simulink model "sst_cllc_ttype_inv"  (R2026a)
settings: Solver=ode23tb  StopTime=simlength  FixedStep=tc  MaxStep=glb_time.tc
values from neighbouring files (symbols this model uses):
  afe_ctrl = ctrl_afe_setup(glb_time.ts_afe, grid_emu.omega_grid_nom)    [init_model.m]
  cllc_ctrl = ctrl_cllc_setup(kp_udc, ki_udc, kp_idc, ki_idc)    [init_model.m]
  glb_time = timing_setup(fpwm_afe, trgo_afe, fpwm_inv, trgo_inv, fpwm_single_phase_inv, trgo_single_phase_inv, fpwm_dab, trgo_dab,      fpwm_psfbc, trgo_psfbc, fpwm_isop_rail, trgo_isop_rail, fpwm_cllc, trgo_cllc, t_measure, tc_factor, tc_decimation, delay_pwm, dead_time_afe,      dead_time_inv, dead_time_single_phase_inv, dead_time_dab, dead_time_psfbc, dead_time_isop_rail, dead_time_cllc)    [init_model.m]
  grid_emu = grid_three_phase_emulator('Dyn11', delta_star, grid_nominal_power, application_voltage, us1, us2, fgrid,                  eq_grid_inductance, eq_grid_resistance, eta, ucc, i1m, p_iron, n1, n2, core_area, core_length, mur,                  up_xi_pu_ref, up_eta_pu_ref, un_xi_pu_ref, un_eta_pu_ref)    [init_model.m]
  lithium_ion_battery_1 = lithium_ion_battery_setup(nominal_battery_voltage_1, nominal_battery_power, initial_battery_soc, glb_time.ts_dab)    [init_model.m]
  omega_set = frequency_set*2*pi    (= 1884.95559215)    [init_model.m]
  single_phase_inverter_ctrl = ctrl_single_phase_inverter_setup(glb_time.ts_inv, pres_ctrl.omega_set,      dqvector_pi.kp_inv, dqvector_pi.ki_inv, pres_ctrl.kp_rpi, pres_ctrl.ki_rpi, pres_ctrl.delta_rpi)    [init_model.m]
  sst_num_of_modules = 2    [init_model.m]
undefined symbols (not defined in the file or in its folder): hwdata
libraries: fl_lib x62, nesl_utility x38, discrete_time_low_pass_filter x8, full_bridge_ideal_switch x4, full_bridge_mosfet_based_with_thermal_model x4, full_bridge_mosfet_based_with_thermal_model_zvs x4, lithium_ion_battery x2, single_phase_transformer x2, dab_single_phase_pwm_modulator x2, dclink_for_three_levels x2, full_bridge_three_level_ttype_ideal_switch_based_model x2, full_bridge_three_level_ttype_mosfet_based_model x2
(part 3 of 5)

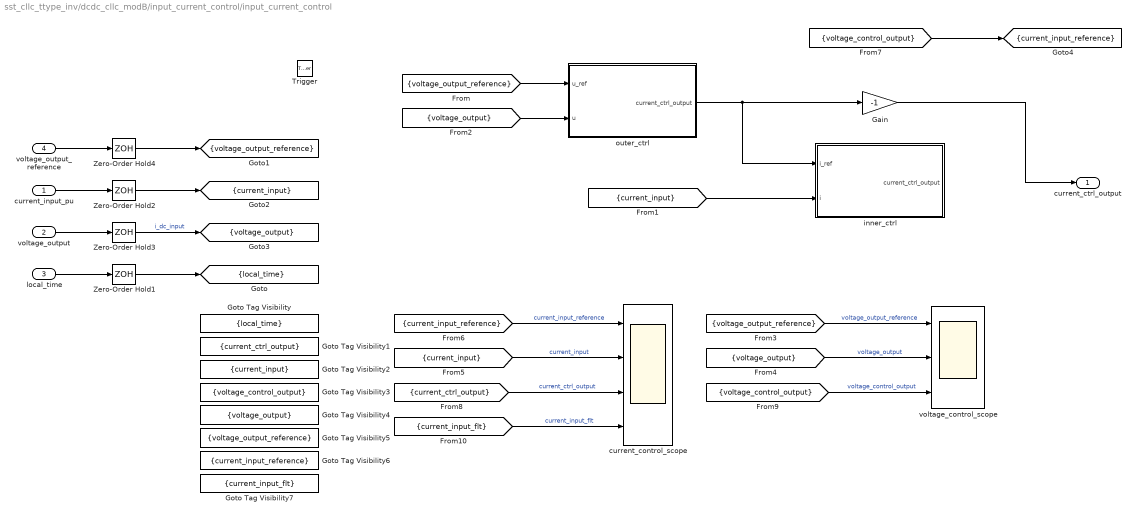
== system sst_cllc_ttype_inv/dcdc_cllc_modB/input_current_control/input_current_control ==
  current_input_pu : Inport
  voltage_output : Inport  Port=2
  local_time : Inport  Port=3
  voltage_output_reference : Inport  Port=4
  Trigger : TriggerPort  VariantControl=(inherit)  PortDimensions=1
  Gain : Gain  Gain=-1
  Goto Tag Visibility : GotoTagVisibility  GotoTag=local_time
  Goto Tag Visibility1 : GotoTagVisibility  GotoTag=current_ctrl_output
  Goto Tag Visibility2 : GotoTagVisibility  GotoTag=current_input
  Goto Tag Visibility3 : GotoTagVisibility  GotoTag=voltage_control_output
  Goto Tag Visibility4 : GotoTagVisibility  GotoTag=voltage_output
  Goto Tag Visibility5 : GotoTagVisibility  GotoTag=voltage_output_reference
  Goto Tag Visibility6 : GotoTagVisibility  GotoTag=current_input_reference
  Goto Tag Visibility7 : GotoTagVisibility  GotoTag=current_input_flt
  Zero-Order Hold{1..4} (4 alike) : ZeroOrderHold  SampleTime=-1
  current_control_scope : Scope  NumInputPorts=4
      settings: ActiveDisplayYMinimum=-0.89123984985351878  ActiveDisplayYMaximum=0.96302534790039185  DataLoggingVariableName=ScopeData12
  inner_ctrl : Subsystem
  outer_ctrl : Subsystem
  voltage_control_scope : Scope  NumInputPorts=3
      settings: ActiveDisplayYMinimum=-2.2572021484375  ActiveDisplayYMaximum=10.3148193359375  DataLoggingVariableName=ScopeData7
  current_ctrl_output : Outport
  tag scope: current_input=scoped, current_input_reference=scoped, local_time=scoped, voltage_output=scoped, voltage_output_reference=scoped
  wires:
  [current_input_flt] -> current_control_scope/4  "current_input_flt"
  [voltage_control_output] -> voltage_control_scope/3  "voltage_control_output"
  [voltage_output] -> voltage_control_scope/2  "voltage_output"
  [voltage_output_reference] -> voltage_control_scope/1  "voltage_output_reference"
  [current_ctrl_output] -> current_control_scope/3  "current_ctrl_output"
  [voltage_control_output] -> [current_input_reference]
  [current_input_reference] -> current_control_scope/1  "current_input_reference"
  [current_input] -> current_control_scope/2  "current_input"
  [voltage_output] -> outer_ctrl/2(u)
  [current_input] -> inner_ctrl/2(i)
  outer_ctrl/1(current_ctrl_output) -> Gain/1, inner_ctrl/1(i_ref)
  [voltage_output_reference] -> outer_ctrl/1(u_ref)
  Zero-Order Hold3/1 -> [voltage_output]  "i_dc_input"
  Zero-Order Hold2/1 -> [current_input]
  Zero-Order Hold4/1 -> [voltage_output_reference]
  voltage_output_reference/1 -> Zero-Order Hold4/1
  Zero-Order Hold1/1 -> [local_time]
  voltage_output/1 -> Zero-Order Hold3/1
  local_time/1 -> Zero-Order Hold1/1
  current_input_pu/1 -> Zero-Order Hold2/1
  Gain/1 -> current_ctrl_output/1

== system sst_cllc_ttype_inv/dcdc_cllc_modB/input_current_control/modulator ==
  phase_displacement : Inport
  Constant1 : Constant  Value=0.5
  Constant2 : Constant  Value=0.5
  dab_single_phase_pwm_modulator : dab_single_phase_pwm_modulator/dab_single_phase_pwm_modulator  fPWM_DAB=glb_time.fPWM_CLLC  m_up=1  m_low=0  dead_time_DAB=glb_time.dead_time_CLLC  pos_cmd_gate=18  neg_cmd_gate=-3  polarity=-1  tc=glb_time.tc  max_phase_displacement=pi/2  trgo_double_update=glb_time.TRGO_CLLC_double_update
  gate_cmds : Outport
  tag scope: TRGO_cllc_modB=global
  wires:
  phase_displacement/1 -> dab_single_phase_pwm_modulator/4
  [time_cllc_module_B] -> dab_single_phase_pwm_modulator/1
  Constant1/1 -> dab_single_phase_pwm_modulator/2
  dab_single_phase_pwm_modulator/1 -> [TRGO_cllc_modB]
  Constant2/1 -> dab_single_phase_pwm_modulator/3
  dab_single_phase_pwm_modulator/2 -> gate_cmds/1

== system sst_cllc_ttype_inv/dcdc_cllc_modB/input_current_control/normalization ==
  in : Inport
  1/Ti3 : Gain  Gain=1/hwdata.cllc.idc1_bez  OutDataTypeStr=double  SaturateOnIntegerOverflow=on  ParamDataTypeStr=Inherit: Same as input
  Quantizer : Quantizer  QuantizationInterval=adc12_quantization
  out_pu : Outport
  wires:
  Quantizer/1 -> out_pu/1
  1/Ti3/1 -> Quantizer/1
  in/1 -> 1/Ti3/1

== system sst_cllc_ttype_inv/dcdc_cllc_modB/input_current_control/normalization1 ==
  in : Inport
  1/Ti3 : Gain  Gain=1/hwdata.cllc.udc2_bez  OutDataTypeStr=double  SaturateOnIntegerOverflow=on  ParamDataTypeStr=Inherit: Same as input
  Quantizer : Quantizer  QuantizationInterval=adc12_quantization
  out_pu : Outport
  wires:
  Quantizer/1 -> out_pu/1
  in/1 -> 1/Ti3/1
  1/Ti3/1 -> Quantizer/1

== system sst_cllc_ttype_inv/single_phase_inverter_modA/dclink/references ==
  m : Inport
  Bus Selector : BusSelector  OutputSignals=udc,udc_p_gnd,udc_n_gnd,Cdc1_current
  Bus Selector1 : BusSelector  OutputSignals=idc1,idc2
  tag scope: CFi_dc_current_modA=global, dclink_n2gnd_voltage_modA=global, dclink_p2gnd_voltage_modA=global, dclink_voltage_modA=global, idc1_m_modA=global, idc2_m_modA=global
  wires:
  m/1 -> Bus Selector/1, Bus Selector1/1
  Bus Selector1/1 -> [idc1_m_modA]  "<idc1>"
  Bus Selector/1 -> [dclink_voltage_modA]  "<udc>"
  Bus Selector/4 -> [CFi_dc_current_modA]  "<Cdc1_current>"
  Bus Selector/3 -> [dclink_n2gnd_voltage_modA]  "<udc_n_gnd>"
  Bus Selector/2 -> [dclink_p2gnd_voltage_modA]  "<udc_p_gnd>"
  Bus Selector1/2 -> [idc2_m_modA]  "<idc2>"

== system sst_cllc_ttype_inv/single_phase_inverter_modA/single phase afe/references ==
  m : Inport
  Bus Selector : BusSelector  OutputSignals=phaseleg_u.mosfet_ploss_Q1,phaseleg_u.mosfet_voltage_Q1,phaseleg_u.mosfet_current_Q1,phaseleg_u.mosfet_JH_temp_Q1,phaseleg_u.mosfet_HA_temp_Q1
  Bus Selector1 : BusSelector  OutputSignals=phaseleg_u.mosfet_ploss_Q2,phaseleg_u.mosfet_voltage_Q2,phaseleg_u.mosfet_current_Q2,phaseleg_u.mosfet_JH_temp_Q2,phaseleg_u.mosfet_HA_temp_Q2
  Bus Selector2 : BusSelector  OutputSignals=phaseleg_u.mosfet_ploss_Q4,phaseleg_u.mosfet_voltage_Q4,phaseleg_u.mosfet_current_Q4,phaseleg_u.mosfet_JH_temp_Q4,phaseleg_u.mosfet_HA_temp_Q4
  Bus Selector3 : BusSelector  OutputSignals=phaseleg_u.mosfet_ploss_Q3,phaseleg_u.mosfet_voltage_Q3,phaseleg_u.mosfet_current_Q3,phaseleg_u.mosfet_JH_temp_Q3,phaseleg_u.mosfet_HA_temp_Q3
  tag scope: mosfet_HA_temp_invQ1=global, mosfet_HA_temp_invQ2=global, mosfet_HA_temp_invQ3=global, mosfet_HA_temp_invQ4=global, mosfet_JH_temp_invQ1=global, mosfet_JH_temp_invQ2=global, mosfet_JH_temp_invQ3=global, mosfet_JH_temp_invQ4=global, mosfet_current_invQ1=global, mosfet_current_invQ2=global, mosfet_current_invQ3=global, mosfet_current_invQ4=global, mosfet_ploss_invQ1=global, mosfet_ploss_invQ2=global, mosfet_ploss_invQ3=global, mosfet_ploss_invQ4=global, mosfet_voltage_invQ1=global, mosfet_voltage_invQ2=global, mosfet_voltage_invQ3=global, mosfet_voltage_invQ4=global
  wires:
  Bus Selector/4 -> [mosfet_JH_temp_invQ1]  "<mosfet_JH_temp_Q1>"
  Bus Selector3/5 -> [mosfet_HA_temp_invQ3]  "<mosfet_HA_temp_Q3>"
  Bus Selector1/1 -> [mosfet_ploss_invQ2]  "<mosfet_ploss_Q2>"
  Bus Selector/5 -> [mosfet_HA_temp_invQ1]  "<mosfet_HA_temp_Q1>"
  Bus Selector/2 -> [mosfet_voltage_invQ1]  "<mosfet_voltage_Q1>"
  Bus Selector2/2 -> [mosfet_voltage_invQ4]  "<mosfet_voltage_Q4>"
  Bus Selector3/3 -> [mosfet_current_invQ3]  "<mosfet_current_Q3>"
  Bus Selector3/2 -> [mosfet_voltage_invQ3]  "<mosfet_voltage_Q3>"
  Bus Selector3/1 -> [mosfet_ploss_invQ3]  "<mosfet_ploss_Q3>"
  Bus Selector2/1 -> [mosfet_ploss_invQ4]  "<mosfet_ploss_Q4>"
  Bus Selector2/5 -> [mosfet_HA_temp_invQ4]  "<mosfet_HA_temp_Q4>"
  m/1 -> Bus Selector2/1, Bus Selector3/1, Bus Selector/1, Bus Selector1/1
  Bus Selector1/2 -> [mosfet_voltage_invQ2]  "<mosfet_voltage_Q2>"
  Bus Selector2/3 -> [mosfet_current_invQ4]  "<mosfet_current_Q4>"
  Bus Selector2/4 -> [mosfet_JH_temp_invQ4]  "<mosfet_JH_temp_Q4>"
  Bus Selector1/4 -> [mosfet_JH_temp_invQ2]  "<mosfet_JH_temp_Q2>"
  Bus Selector/1 -> [mosfet_ploss_invQ1]  "<mosfet_ploss_Q1>"
  Bus Selector1/3 -> [mosfet_current_invQ2]  "<mosfet_current_Q2>"
  Bus Selector3/4 -> [mosfet_JH_temp_invQ3]  "<mosfet_JH_temp_Q3>"
  Bus Selector/3 -> [mosfet_current_invQ1]  "<mosfet_current_Q1>"
  Bus Selector1/5 -> [mosfet_HA_temp_invQ2]  "<mosfet_HA_temp_Q2>"

== system sst_cllc_ttype_inv/single_phase_inverter_modA/single phase inverter control/acquisition_and_scaling_current ==
  in : Inport
  1/Ti5 : Gain  Gain=1/hwdata.single_phase_inverter.ibez  SaturateOnIntegerOverflow=on  OutDataTypeStr=Inherit: Same as input  ParamDataTypeStr=Inherit: Same as input
  Quantizer : Quantizer  QuantizationInterval=adc11_quantization
  out : Outport
  wires:
  Quantizer/1 -> out/1
  1/Ti5/1 -> Quantizer/1
  in/1 -> 1/Ti5/1

== system sst_cllc_ttype_inv/single_phase_inverter_modA/single phase inverter control/acquisition_and_scaling_current_with_white_noise ==
  in : Inport
  1/Ti5 : Gain  Gain=1/hwdata.single_phase_inverter.ibez  SaturateOnIntegerOverflow=on  OutDataTypeStr=Inherit: Same as input  ParamDataTypeStr=Inherit: Same as input
  Band-Limited White Noise : simulink/Sources/Band-Limited White Noise  Commented=on  Cov=1e-10  Ts=glb_time.tc  seed=[23341]
  Quantizer : Quantizer  QuantizationInterval=adc12_quantization
  Sum : Sum  Inputs=|++
  current_measure_with-without noise : Scope  NumInputPorts=2
      settings: ActiveDisplayYMinimum=-42.907449410116151  ActiveDisplayYMaximum=14.197534402303543  DataLoggingVariableName=ScopeData15
  out : Outport
  wires:
  1/Ti5/1 -> current_measure_with-without noise/1, Sum/1  "iload_without_noise"
  Sum/1 -> Quantizer/1
  Band-Limited White Noise/1 -> Sum/2
  Quantizer/1 -> out/1, current_measure_with-without noise/2  "iload_with_noise"
  in/1 -> 1/Ti5/1

== system sst_cllc_ttype_inv/single_phase_inverter_modA/single phase inverter control/acquisition_and_scaling_dc_voltage ==
  in : Inport
  1/Ti3 : Gain  Gain=1/hwdata.single_phase_inverter.udc_nom  SaturateOnIntegerOverflow=on  OutDataTypeStr=Inherit: Same as input  ParamDataTypeStr=Inherit: Same as input
  Quantizer : Quantizer  QuantizationInterval=adc12_quantization
  out : Outport
  wires:
  in/1 -> 1/Ti3/1
  1/Ti3/1 -> Quantizer/1
  Quantizer/1 -> out/1

== system sst_cllc_ttype_inv/single_phase_inverter_modA/single phase inverter control/acquisition_and_scaling_grid_voltage_ac ==
  in : Inport
  1/Ti1 : Gain  Gain=sst_num_of_modules  SaturateOnIntegerOverflow=on  OutDataTypeStr=Inherit: Same as input  ParamDataTypeStr=Inherit: Same as input
  1/Ti5 : Gain  Gain=1/grid_emu.u2bez  SaturateOnIntegerOverflow=on  OutDataTypeStr=Inherit: Same as input  ParamDataTypeStr=Inherit: Same as input
  Quantizer : Quantizer  QuantizationInterval=adc12_quantization
  out : Outport
  wires:
  Quantizer/1 -> out/1
  1/Ti5/1 -> Quantizer/1
  in/1 -> 1/Ti1/1
  1/Ti1/1 -> 1/Ti5/1

== system sst_cllc_ttype_inv/single_phase_inverter_modA/single phase inverter control/acquisition_and_scaling_voltage ==
  in : Inport
  1/Ti5 : Gain  Gain=1/hwdata.single_phase_inverter.ubez  SaturateOnIntegerOverflow=on  OutDataTypeStr=Inherit: Same as input  ParamDataTypeStr=Inherit: Same as input
  Quantizer : Quantizer  QuantizationInterval=adc12_quantization
  pwm filtering for measure : cstblocks_lti/LTI System  sys=sogi.flt.beta  IC=[]  PadeOrder=0
  out : Outport
  wires:
  in/1 -> 1/Ti5/1
  pwm filtering for measure/1 -> Quantizer/1
  1/Ti5/1 -> pwm filtering for measure/1
  Quantizer/1 -> out/1

== system sst_cllc_ttype_inv/single_phase_inverter_modA/single phase inverter control/inverter_current_output_pu_reference ==
  Rate Limiter : RateLimiter  RisingSlewLimit=2  FallingSlewLimit=-2  SampleTimeMode=inherited
  Step : Step  Time=0.35  SampleTime=0
  afe_current_output_pu_reference : Outport
  wires:
  Step/1 -> Rate Limiter/1
  Rate Limiter/1 -> afe_current_output_pu_reference/1

== system sst_cllc_ttype_inv/single_phase_inverter_modA/single phase inverter control/pwm modulator ==
  vout : Inport
  Constant : Constant  Value=0
  single_phase_three_levels_PWM_generator_with_global_TRGO : single_phase_three_levels_PWM_modulator/single_phase_three_levels_PWM_generator_with_global_TRGO  f=glb_time.fPWM_INV  m_up=1  m_low=-1  dead_time=glb_time.dead_time_AFE  pos_cmd_gate=15  neg_cmd_gate=-10  polarity=1  tc=glb_time.tc  double_sampling=glb_time.TRGO_AFE_double_update
  gate_cmds : Outport
  tag scope: TRGO_AFE_modA=global
  wires:
  vout/1 -> single_phase_three_levels_PWM_generator_with_global_TRGO/3
  Constant/1 -> single_phase_three_levels_PWM_generator_with_global_TRGO/2
  single_phase_three_levels_PWM_generator_with_global_TRGO/2 -> gate_cmds/1
  single_phase_three_levels_PWM_generator_with_global_TRGO/1 -> [TRGO_AFE_modA]
  [time_afe_module_A] -> single_phase_three_levels_PWM_generator_with_global_TRGO/1

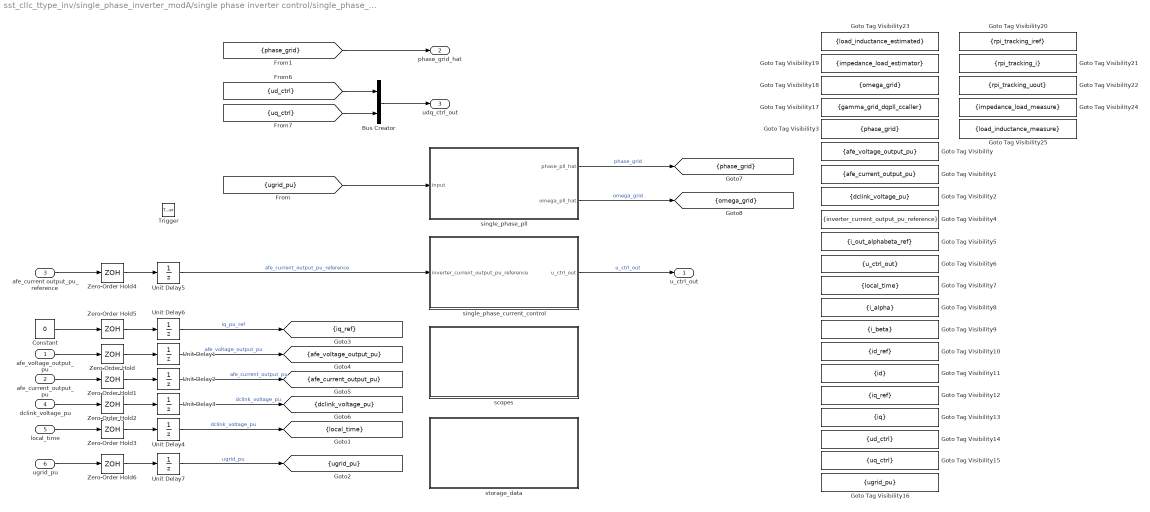
== system sst_cllc_ttype_inv/single_phase_inverter_modA/single phase inverter control/single_phase_inverter_ctrl ==
  afe_voltage_output_pu : Inport
  afe_current_output_pu : Inport  Port=2
  afe_current output_pu_reference : Inport  Port=3
  dclink_voltage_pu : Inport  Port=4
  local_time : Inport  Port=5
  ugrid_pu : Inport  Port=6
  Trigger : TriggerPort  VariantControl=(inherit)  PortDimensions=1
  Bus Creator : BusCreator  Inputs=2
  Constant : Constant  Value=0
  Goto Tag Visibility : GotoTagVisibility  GotoTag=afe_voltage_output_pu
  Goto Tag Visibility1 : GotoTagVisibility  GotoTag=afe_current_output_pu
  Goto Tag Visibility10 : GotoTagVisibility  GotoTag=id_ref
  Goto Tag Visibility11 : GotoTagVisibility  GotoTag=id
  Goto Tag Visibility12 : GotoTagVisibility  GotoTag=iq_ref
  Goto Tag Visibility13 : GotoTagVisibility  GotoTag=iq
  Goto Tag Visibility14 : GotoTagVisibility  GotoTag=ud_ctrl
  Goto Tag Visibility15 : GotoTagVisibility  GotoTag=uq_ctrl
  Goto Tag Visibility16 : GotoTagVisibility  GotoTag=ugrid_pu
  Goto Tag Visibility17 : GotoTagVisibility  GotoTag=gamma_grid_dqpll_ccaller
  Goto Tag Visibility18 : GotoTagVisibility  GotoTag=omega_grid
  Goto Tag Visibility19 : GotoTagVisibility  GotoTag=impedance_load_estimator
  Goto Tag Visibility2 : GotoTagVisibility  GotoTag=dclink_voltage_pu
  Goto Tag Visibility20 : GotoTagVisibility  GotoTag=rpi_tracking_iref
  Goto Tag Visibility21 : GotoTagVisibility  GotoTag=rpi_tracking_i
  Goto Tag Visibility22 : GotoTagVisibility  GotoTag=rpi_tracking_uout
  Goto Tag Visibility23 : GotoTagVisibility  GotoTag=load_inductance_estimated
  Goto Tag Visibility24 : GotoTagVisibility  GotoTag=impedance_load_measure
  Goto Tag Visibility25 : GotoTagVisibility  GotoTag=load_inductance_measure
  Goto Tag Visibility3 : GotoTagVisibility  GotoTag=phase_grid
  Goto Tag Visibility4 : GotoTagVisibility  GotoTag=inverter_current_output_pu_reference
  Goto Tag Visibility5 : GotoTagVisibility  GotoTag=i_out_alphabeta_ref
  Goto Tag Visibility6 : GotoTagVisibility  GotoTag=u_ctrl_out
  Goto Tag Visibility7 : GotoTagVisibility  GotoTag=local_time
  Goto Tag Visibility8 : GotoTagVisibility  GotoTag=i_alpha
  Goto Tag Visibility9 : GotoTagVisibility  GotoTag=i_beta
  Unit Delay{1..7} (7 alike) : UnitDelay  SampleTime=-1
  Zero-Order Hold{,1..6} (7 alike) : ZeroOrderHold  SampleTime=-1
  scopes : Subsystem
  single_phase_current_control : Subsystem
  single_phase_pll : Subsystem
  storage_data : Subsystem
  u_ctrl_out : Outport
  phase_grid_hat : Outport  Port=2
  udq_ctrl_out : Outport  Port=3
  tag scope: afe_current_output_pu=scoped, afe_voltage_output_pu=scoped, dclink_voltage_pu=scoped, iq_ref=scoped, local_time=scoped, omega_grid=scoped, phase_grid=scoped, ugrid_pu=scoped
  wires:
  afe_voltage_output_pu/1 -> Zero-Order Hold/1
  afe_current_output_pu/1 -> Zero-Order Hold1/1
  dclink_voltage_pu/1 -> Zero-Order Hold2/1
  Unit Delay1/1 -> [afe_voltage_output_pu]  "afe_voltage_output_pu"
  Unit Delay2/1 -> [afe_current_output_pu]  "afe_current_output_pu"
  Unit Delay3/1 -> [dclink_voltage_pu]  "dclink_voltage_pu"
  single_phase_pll/1(phase_pll_hat) -> [phase_grid]  "phase_grid"
  afe_current output_pu_reference/1 -> Zero-Order Hold4/1
  single_phase_current_control/1(u_ctrl_out) -> u_ctrl_out/1  "u_ctrl_out"
  Zero-Order Hold/1 -> Unit Delay1/1
  Zero-Order Hold1/1 -> Unit Delay2/1
  Zero-Order Hold2/1 -> Unit Delay3/1
  Zero-Order Hold3/1 -> Unit Delay4/1
  Unit Delay4/1 -> [local_time]  "dclink_voltage_pu"
  local_time/1 -> Zero-Order Hold3/1
  Zero-Order Hold4/1 -> Unit Delay5/1
  Unit Delay5/1 -> single_phase_current_control/1(inverter_current_output_pu_reference)  "afe_current_output_pu_reference"
  Constant/1 -> Zero-Order Hold5/1
  Zero-Order Hold5/1 -> Unit Delay6/1
  Unit Delay6/1 -> [iq_ref]  "iq_pu_ref"
  ugrid_pu/1 -> Zero-Order Hold6/1
  Zero-Order Hold6/1 -> Unit Delay7/1
  Unit Delay7/1 -> [ugrid_pu]  "ugrid_pu"
  single_phase_pll/2(omega_pll_hat) -> [omega_grid]  "omega_grid"
  [ugrid_pu] -> single_phase_pll/1(input)
  [phase_grid] -> phase_grid_hat/1
  Bus Creator/1 -> udq_ctrl_out/1
  [ud_ctrl] -> Bus Creator/1
  [uq_ctrl] -> Bus Creator/2

== system sst_cllc_ttype_inv/single_phase_inverter_modB/dclink/references ==
  m : Inport
  Bus Selector : BusSelector  OutputSignals=udc,udc_p_gnd,udc_n_gnd,Cdc1_current
  Bus Selector1 : BusSelector  OutputSignals=idc1,idc2
  tag scope: CFi_dc_current_modB=global, dclink_n2gnd_voltage_modB=global, dclink_p2gnd_voltage_modB=global, dclink_voltage_modB=global, idc1_m_modB=global, idc2_m_modB=global
  wires:
  Bus Selector1/2 -> [idc2_m_modB]  "<idc2>"
  Bus Selector/2 -> [dclink_p2gnd_voltage_modB]  "<udc_p_gnd>"
  Bus Selector/3 -> [dclink_n2gnd_voltage_modB]  "<udc_n_gnd>"
  Bus Selector/4 -> [CFi_dc_current_modB]  "<Cdc1_current>"
  Bus Selector/1 -> [dclink_voltage_modB]  "<udc>"
  Bus Selector1/1 -> [idc1_m_modB]  "<idc1>"
  m/1 -> Bus Selector1/1, Bus Selector/1

== system sst_cllc_ttype_inv/single_phase_inverter_modB/single phase afe/references ==
  m : Inport
  Bus Selector : BusSelector  OutputSignals=phaseleg_u.mosfet_ploss_Q1,phaseleg_u.mosfet_voltage_Q1,phaseleg_u.mosfet_current_Q1,phaseleg_u.mosfet_JH_temp_Q1,phaseleg_u.mosfet_HA_temp_Q1
  Bus Selector1 : BusSelector  OutputSignals=phaseleg_u.mosfet_ploss_Q2,phaseleg_u.mosfet_voltage_Q2,phaseleg_u.mosfet_current_Q2,phaseleg_u.mosfet_JH_temp_Q2,phaseleg_u.mosfet_HA_temp_Q2
  Bus Selector2 : BusSelector  OutputSignals=phaseleg_u.mosfet_ploss_Q4,phaseleg_u.mosfet_voltage_Q4,phaseleg_u.mosfet_current_Q4,phaseleg_u.mosfet_JH_temp_Q4,phaseleg_u.mosfet_HA_temp_Q4
  Bus Selector3 : BusSelector  OutputSignals=phaseleg_u.mosfet_ploss_Q3,phaseleg_u.mosfet_voltage_Q3,phaseleg_u.mosfet_current_Q3,phaseleg_u.mosfet_JH_temp_Q3,phaseleg_u.mosfet_HA_temp_Q3
  tag scope: mosfet_HA_temp_invQ1=global, mosfet_HA_temp_invQ2=global, mosfet_HA_temp_invQ3=global, mosfet_HA_temp_invQ4=global, mosfet_JH_temp_invQ1=global, mosfet_JH_temp_invQ2=global, mosfet_JH_temp_invQ3=global, mosfet_JH_temp_invQ4=global, mosfet_current_invQ1=global, mosfet_current_invQ2=global, mosfet_current_invQ3=global, mosfet_current_invQ4=global, mosfet_ploss_invQ1=global, mosfet_ploss_invQ2=global, mosfet_ploss_invQ3=global, mosfet_ploss_invQ4=global, mosfet_voltage_invQ1=global, mosfet_voltage_invQ2=global, mosfet_voltage_invQ3=global, mosfet_voltage_invQ4=global
  wires:
  Bus Selector1/5 -> [mosfet_HA_temp_invQ2]  "<mosfet_HA_temp_Q2>"
  Bus Selector/3 -> [mosfet_current_invQ1]  "<mosfet_current_Q1>"
  Bus Selector3/4 -> [mosfet_JH_temp_invQ3]  "<mosfet_JH_temp_Q3>"
  Bus Selector1/3 -> [mosfet_current_invQ2]  "<mosfet_current_Q2>"
  Bus Selector/1 -> [mosfet_ploss_invQ1]  "<mosfet_ploss_Q1>"
  Bus Selector1/4 -> [mosfet_JH_temp_invQ2]  "<mosfet_JH_temp_Q2>"
  Bus Selector2/4 -> [mosfet_JH_temp_invQ4]  "<mosfet_JH_temp_Q4>"
  Bus Selector2/3 -> [mosfet_current_invQ4]  "<mosfet_current_Q4>"
  Bus Selector1/2 -> [mosfet_voltage_invQ2]  "<mosfet_voltage_Q2>"
  m/1 -> Bus Selector1/1, Bus Selector/1, Bus Selector3/1, Bus Selector2/1
  Bus Selector2/5 -> [mosfet_HA_temp_invQ4]  "<mosfet_HA_temp_Q4>"
  Bus Selector2/1 -> [mosfet_ploss_invQ4]  "<mosfet_ploss_Q4>"
  Bus Selector3/1 -> [mosfet_ploss_invQ3]  "<mosfet_ploss_Q3>"
  Bus Selector3/2 -> [mosfet_voltage_invQ3]  "<mosfet_voltage_Q3>"
  Bus Selector3/3 -> [mosfet_current_invQ3]  "<mosfet_current_Q3>"
  Bus Selector2/2 -> [mosfet_voltage_invQ4]  "<mosfet_voltage_Q4>"
  Bus Selector/2 -> [mosfet_voltage_invQ1]  "<mosfet_voltage_Q1>"
  Bus Selector/5 -> [mosfet_HA_temp_invQ1]  "<mosfet_HA_temp_Q1>"
  Bus Selector1/1 -> [mosfet_ploss_invQ2]  "<mosfet_ploss_Q2>"
  Bus Selector3/5 -> [mosfet_HA_temp_invQ3]  "<mosfet_HA_temp_Q3>"
  Bus Selector/4 -> [mosfet_JH_temp_invQ1]  "<mosfet_JH_temp_Q1>"

== system sst_cllc_ttype_inv/single_phase_inverter_modB/single phase inverter control/acquisition_and_scaling_current_with_white_noise ==
  in : Inport
  1/Ti5 : Gain  Gain=1/hwdata.single_phase_inverter.ibez  SaturateOnIntegerOverflow=on  OutDataTypeStr=Inherit: Same as input  ParamDataTypeStr=Inherit: Same as input
  Band-Limited White Noise : simulink/Sources/Band-Limited White Noise  Commented=on  Cov=1e-10  Ts=glb_time.tc  seed=[23341]
  Quantizer : Quantizer  QuantizationInterval=adc12_quantization
  Sum : Sum  Inputs=|++
  current_measure_with-without noise : Scope  NumInputPorts=2
      settings: ActiveDisplayYMinimum=-42.907449410116151  ActiveDisplayYMaximum=14.197534402303543  DataLoggingVariableName=ScopeData15
  out : Outport
  wires:
  in/1 -> 1/Ti5/1
  Quantizer/1 -> current_measure_with-without noise/2, out/1  "iload_with_noise"
  Band-Limited White Noise/1 -> Sum/2
  Sum/1 -> Quantizer/1
  1/Ti5/1 -> Sum/1, current_measure_with-without noise/1  "iload_without_noise"

== system sst_cllc_ttype_inv/single_phase_inverter_modB/single phase inverter control/acquisition_and_scaling_dc_voltage ==
  in : Inport
  1/Ti3 : Gain  Gain=1/hwdata.single_phase_inverter.udc_nom  SaturateOnIntegerOverflow=on  OutDataTypeStr=Inherit: Same as input  ParamDataTypeStr=Inherit: Same as input
  Quantizer : Quantizer  QuantizationInterval=adc12_quantization
  out : Outport
  wires:
  Quantizer/1 -> out/1
  1/Ti3/1 -> Quantizer/1
  in/1 -> 1/Ti3/1

== system sst_cllc_ttype_inv/single_phase_inverter_modB/single phase inverter control/acquisition_and_scaling_grid_voltage_ac ==
  in : Inport
  1/Ti1 : Gain  Gain=sst_num_of_modules  SaturateOnIntegerOverflow=on  OutDataTypeStr=Inherit: Same as input  ParamDataTypeStr=Inherit: Same as input
  1/Ti5 : Gain  Gain=1/grid_emu.u2bez  SaturateOnIntegerOverflow=on  OutDataTypeStr=Inherit: Same as input  ParamDataTypeStr=Inherit: Same as input
  Quantizer : Quantizer  QuantizationInterval=adc12_quantization
  out : Outport
  wires:
  in/1 -> 1/Ti1/1
  1/Ti5/1 -> Quantizer/1
  Quantizer/1 -> out/1
  1/Ti1/1 -> 1/Ti5/1

== system sst_cllc_ttype_inv/single_phase_inverter_modB/single phase inverter control/acquisition_and_scaling_voltage ==
  in : Inport
  1/Ti5 : Gain  Gain=1/hwdata.single_phase_inverter.ubez  SaturateOnIntegerOverflow=on  OutDataTypeStr=Inherit: Same as input  ParamDataTypeStr=Inherit: Same as input
  Quantizer : Quantizer  QuantizationInterval=adc12_quantization
  pwm filtering for measure : cstblocks_lti/LTI System  sys=sogi.flt.beta  IC=[]  PadeOrder=0
  out : Outport
  wires:
  Quantizer/1 -> out/1
  1/Ti5/1 -> pwm filtering for measure/1
  pwm filtering for measure/1 -> Quantizer/1
  in/1 -> 1/Ti5/1

== system sst_cllc_ttype_inv/single_phase_inverter_modB/single phase inverter control/inverter_current_output_pu_reference ==
  Constant : Constant  Value=0.5
  afe_current_output_pu_reference : Outport
  wires:
  Constant/1 -> afe_current_output_pu_reference/1

== system sst_cllc_ttype_inv/single_phase_inverter_modB/single phase inverter control/pwm modulator ==
  vout : Inport
  Constant : Constant  Value=0
  single_phase_three_levels_PWM_generator_with_global_TRGO : single_phase_three_levels_PWM_modulator/single_phase_three_levels_PWM_generator_with_global_TRGO  f=glb_time.fPWM_INV  m_up=1  m_low=-1  dead_time=glb_time.dead_time_AFE  pos_cmd_gate=15  neg_cmd_gate=-10  polarity=1  tc=glb_time.tc  double_sampling=glb_time.TRGO_AFE_double_update
  gate_cmds : Outport
  tag scope: TRGO_AFE_modB=global
  wires:
  [time_afe_module_B] -> single_phase_three_levels_PWM_generator_with_global_TRGO/1
  single_phase_three_levels_PWM_generator_with_global_TRGO/1 -> [TRGO_AFE_modB]
  single_phase_three_levels_PWM_generator_with_global_TRGO/2 -> gate_cmds/1
  Constant/1 -> single_phase_three_levels_PWM_generator_with_global_TRGO/2
  vout/1 -> single_phase_three_levels_PWM_generator_with_global_TRGO/3

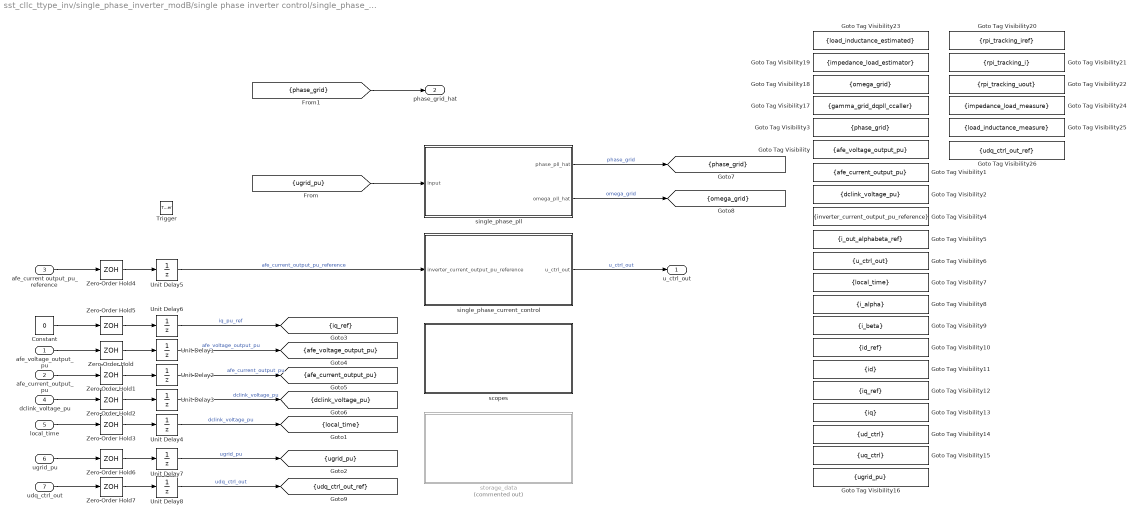
== system sst_cllc_ttype_inv/single_phase_inverter_modB/single phase inverter control/single_phase_inverter_ctrl ==
  afe_voltage_output_pu : Inport
  afe_current_output_pu : Inport  Port=2
  afe_current output_pu_reference : Inport  Port=3
  dclink_voltage_pu : Inport  Port=4
  local_time : Inport  Port=5
  ugrid_pu : Inport  Port=6
  udq_ctrl_out : Inport  Port=7
  Trigger : TriggerPort  VariantControl=(inherit)  PortDimensions=1
  Constant : Constant  Value=0
  Goto Tag Visibility : GotoTagVisibility  GotoTag=afe_voltage_output_pu
  Goto Tag Visibility1 : GotoTagVisibility  GotoTag=afe_current_output_pu
  Goto Tag Visibility10 : GotoTagVisibility  GotoTag=id_ref
  Goto Tag Visibility11 : GotoTagVisibility  GotoTag=id
  Goto Tag Visibility12 : GotoTagVisibility  GotoTag=iq_ref
  Goto Tag Visibility13 : GotoTagVisibility  GotoTag=iq
  Goto Tag Visibility14 : GotoTagVisibility  GotoTag=ud_ctrl
  Goto Tag Visibility15 : GotoTagVisibility  GotoTag=uq_ctrl
  Goto Tag Visibility16 : GotoTagVisibility  GotoTag=ugrid_pu
  Goto Tag Visibility17 : GotoTagVisibility  GotoTag=gamma_grid_dqpll_ccaller
  Goto Tag Visibility18 : GotoTagVisibility  GotoTag=omega_grid
  Goto Tag Visibility19 : GotoTagVisibility  GotoTag=impedance_load_estimator
  Goto Tag Visibility2 : GotoTagVisibility  GotoTag=dclink_voltage_pu
  Goto Tag Visibility20 : GotoTagVisibility  GotoTag=rpi_tracking_iref
  Goto Tag Visibility21 : GotoTagVisibility  GotoTag=rpi_tracking_i
  Goto Tag Visibility22 : GotoTagVisibility  GotoTag=rpi_tracking_uout
  Goto Tag Visibility23 : GotoTagVisibility  GotoTag=load_inductance_estimated
  Goto Tag Visibility24 : GotoTagVisibility  GotoTag=impedance_load_measure
  Goto Tag Visibility25 : GotoTagVisibility  GotoTag=load_inductance_measure
  Goto Tag Visibility26 : GotoTagVisibility  GotoTag=udq_ctrl_out_ref
  Goto Tag Visibility3 : GotoTagVisibility  GotoTag=phase_grid
  Goto Tag Visibility4 : GotoTagVisibility  GotoTag=inverter_current_output_pu_reference
  Goto Tag Visibility5 : GotoTagVisibility  GotoTag=i_out_alphabeta_ref
  Goto Tag Visibility6 : GotoTagVisibility  GotoTag=u_ctrl_out
  Goto Tag Visibility7 : GotoTagVisibility  GotoTag=local_time
  Goto Tag Visibility8 : GotoTagVisibility  GotoTag=i_alpha
  Goto Tag Visibility9 : GotoTagVisibility  GotoTag=i_beta
  Unit Delay{1..8} (8 alike) : UnitDelay  SampleTime=-1
  Zero-Order Hold{,1..7} (8 alike) : ZeroOrderHold  SampleTime=-1
  scopes : Subsystem
  single_phase_current_control : Subsystem
  single_phase_pll : Subsystem
  storage_data : Subsystem  Commented=on
  u_ctrl_out : Outport
  phase_grid_hat : Outport  Port=2
  tag scope: afe_current_output_pu=scoped, afe_voltage_output_pu=scoped, dclink_voltage_pu=scoped, iq_ref=scoped, local_time=scoped, omega_grid=scoped, phase_grid=scoped, udq_ctrl_out_ref=scoped, ugrid_pu=scoped
  wires:
  [phase_grid] -> phase_grid_hat/1
  [ugrid_pu] -> single_phase_pll/1(input)
  single_phase_pll/2(omega_pll_hat) -> [omega_grid]  "omega_grid"
  Unit Delay7/1 -> [ugrid_pu]  "ugrid_pu"
  Zero-Order Hold6/1 -> Unit Delay7/1
  ugrid_pu/1 -> Zero-Order Hold6/1
  Unit Delay6/1 -> [iq_ref]  "iq_pu_ref"
  Zero-Order Hold5/1 -> Unit Delay6/1
  Constant/1 -> Zero-Order Hold5/1
  Unit Delay5/1 -> single_phase_current_control/1(inverter_current_output_pu_reference)  "afe_current_output_pu_reference"
  Zero-Order Hold4/1 -> Unit Delay5/1
  local_time/1 -> Zero-Order Hold3/1
  Unit Delay4/1 -> [local_time]  "dclink_voltage_pu"
  Zero-Order Hold3/1 -> Unit Delay4/1
  Zero-Order Hold2/1 -> Unit Delay3/1
  Zero-Order Hold1/1 -> Unit Delay2/1
  Zero-Order Hold/1 -> Unit Delay1/1
  single_phase_current_control/1(u_ctrl_out) -> u_ctrl_out/1  "u_ctrl_out"
  afe_current output_pu_reference/1 -> Zero-Order Hold4/1
  single_phase_pll/1(phase_pll_hat) -> [phase_grid]  "phase_grid"
  Unit Delay3/1 -> [dclink_voltage_pu]  "dclink_voltage_pu"
  Unit Delay2/1 -> [afe_current_output_pu]  "afe_current_output_pu"
  Unit Delay1/1 -> [afe_voltage_output_pu]  "afe_voltage_output_pu"
  dclink_voltage_pu/1 -> Zero-Order Hold2/1
  afe_current_output_pu/1 -> Zero-Order Hold1/1
  afe_voltage_output_pu/1 -> Zero-Order Hold/1
  udq_ctrl_out/1 -> Zero-Order Hold7/1
  Zero-Order Hold7/1 -> Unit Delay8/1
  Unit Delay8/1 -> [udq_ctrl_out_ref]  "udq_ctrl_out"

== system sst_cllc_ttype_inv/dcdc_cllc_modA/dcdc_with_galvanic_isolation/full-bridge_1/full-bridge_ideal_switch_based ==
  gate_commands : Inport
  data_measure : Subsystem
  full-bridge_ideal_switch_based : full_bridge_ideal_switch/full-bridge ideal switch based  Rds_on=ideal_switch.dab.Rds_on  Vdon_diode=ideal_switch.dab.Vdon_diode  Rdon_diode=ideal_switch.dab.Rdon_diode  Csnubber=ideal_switch.dab.Csnubber_zvs  Rsnubber=ideal_switch.dab.Rsnubber_zvs  Vth=ideal_switch.dab.Vth
  udc(+) : PMIOPort  Side=Left
  uac(+) : PMIOPort  Port=2  Side=Right
  udc(-) : PMIOPort  Port=3  Side=Left
  uac(-) : PMIOPort  Port=4  Side=Right
  wires:
  full-bridge_ideal_switch_based/1 -> data_measure/1(m)
  gate_commands/1 -> full-bridge_ideal_switch_based/1
  connections:
  udc(+)/RConn1 -- full-bridge_ideal_switch_based/LConn1
  udc(-)/RConn1 -- full-bridge_ideal_switch_based/LConn2
  full-bridge_ideal_switch_based/RConn1 -- uac(+)/RConn1
  uac(-)/RConn1 -- full-bridge_ideal_switch_based/RConn2

== system sst_cllc_ttype_inv/dcdc_cllc_modA/dcdc_with_galvanic_isolation/full-bridge_1/full-bridge_mosfet_based_with_thermal_model ==
  gate_commands : Inport
  data_measure : Subsystem
  full-bridge_mosfet_based_with_thermal_model : full_bridge_mosfet_based_with_thermal_model/full-bridge mosfet based with thermal model  mass_heatsink_m=heatsink.no_weight  specific_heat_m=heatsink.cp  rth_mosfet_HA_m=heatsink.Rth_mosfet_HA  rth_mosfet_JH_m=mosfet.dab.Rth_mosfet_JH  Rds_on_m=mosfet.dab.Rds_on  Vth_m=mosfet.dab.Vth  Eon_m=mosfet.dab.Eon  Eoff_m=mosfet.dab.Eoff  Voff_sw_loss_m=mosfet.dab.Voff_sw_losses  Ion_sw_loss_m=mosfet.dab.Ion_sw_losses  Vdon_diode_m=mosfet.dab.Vdon_diode  Rdon_diode_m=mosfet.dab.Rds_on  JunctionTermalMass_m=mosfet.dab.JunctionTermalMass  Tambient_m=heatsink.Tambient  DThs_init_m=heatsink.DThs_init
  udc(+) : PMIOPort  Side=Left
  uac(+) : PMIOPort  Port=2  Side=Right
  udc(-) : PMIOPort  Port=3  Side=Left
  uac(-) : PMIOPort  Port=4  Side=Right
  wires:
  full-bridge_mosfet_based_with_thermal_model/1 -> data_measure/1(m)
  gate_commands/1 -> full-bridge_mosfet_based_with_thermal_model/1
  connections:
  full-bridge_mosfet_based_with_thermal_model/RConn2 -- uac(-)/RConn1
  full-bridge_mosfet_based_with_thermal_model/LConn1 -- udc(+)/RConn1
  udc(-)/RConn1 -- full-bridge_mosfet_based_with_thermal_model/LConn2
  full-bridge_mosfet_based_with_thermal_model/RConn1 -- uac(+)/RConn1

== system sst_cllc_ttype_inv/dcdc_cllc_modA/dcdc_with_galvanic_isolation/full-bridge_1/full-bridge_mosfet_based_with_thermal_model_zvs ==
  gate_commands : Inport
  data_measure : Subsystem
  full-bridge_mosfet_based_ with_thermal_model_zvs : full_bridge_mosfet_based_with_thermal_model_zvs/full-bridge_mosfet_based_ with_thermal_model_zvs  mass_heatsink_m=heatsink.no_weight  specific_heat_m=heatsink.cp  rth_mosfet_HA_m=heatsink.Rth_mosfet_HA  rth_mosfet_JH_m=mosfet.dab.Rth_mosfet_JH  Rds_on_m=mosfet.dab.Rds_on  Vth_m=mosfet.dab.Vth  Eon_m=mosfet.dab.Eon  Eoff_m=mosfet.dab.Eoff  Voff_sw_loss_m=mosfet.dab.Voff_sw_losses  Ion_sw_loss_m=mosfet.dab.Ion_sw_losses  Vdon_diode_m=mosfet.dab.Vdon_diode  Rdon_diode_m=mosfet.dab.Rds_on  JunctionTermalMass_m=mosfet.dab.JunctionTermalMass  Tambient_m=heatsink.Tambient  DThs_init_m=heatsink.DThs_init  Csnubber_m=mosfet.dab.Csnubber_zvs  Rsnubber_m=mosfet.dab.Rsnubber_zvs
  udc(+) : PMIOPort  Side=Left
  udc(-) : PMIOPort  Port=2  Side=Left
  uac(+) : PMIOPort  Port=3  Side=Right
  uac(-) : PMIOPort  Port=4  Side=Right
  wires:
  full-bridge_mosfet_based_ with_thermal_model_zvs/1 -> data_measure/1(m)
  gate_commands/1 -> full-bridge_mosfet_based_ with_thermal_model_zvs/1
  connections:
  full-bridge_mosfet_based_ with_thermal_model_zvs/LConn2 -- udc(-)/RConn1
  full-bridge_mosfet_based_ with_thermal_model_zvs/LConn1 -- udc(+)/RConn1
  full-bridge_mosfet_based_ with_thermal_model_zvs/RConn2 -- uac(-)/RConn1
  full-bridge_mosfet_based_ with_thermal_model_zvs/RConn1 -- uac(+)/RConn1

== system sst_cllc_ttype_inv/dcdc_cllc_modA/dcdc_with_galvanic_isolation/full-bridge_2/full-bridge_ideal_switch_based ==
  gate_commands : Inport
  data_measure : Subsystem
  full-bridge_ideal_switch_based : full_bridge_ideal_switch/full-bridge ideal switch based  Rds_on=ideal_switch.dab.Rds_on  Vdon_diode=ideal_switch.dab.Vdon_diode  Rdon_diode=ideal_switch.dab.Rdon_diode  Csnubber=ideal_switch.dab.Csnubber_zvs  Rsnubber=ideal_switch.dab.Rsnubber_zvs  Vth=ideal_switch.dab.Vth
  udc(+) : PMIOPort  Side=Left
  uac(+) : PMIOPort  Port=2  Side=Right
  udc(-) : PMIOPort  Port=3  Side=Left
  uac(-) : PMIOPort  Port=4  Side=Right
  wires:
  full-bridge_ideal_switch_based/1 -> data_measure/1(m)
  gate_commands/1 -> full-bridge_ideal_switch_based/1
  connections:
  udc(+)/RConn1 -- full-bridge_ideal_switch_based/LConn1
  udc(-)/RConn1 -- full-bridge_ideal_switch_based/LConn2
  full-bridge_ideal_switch_based/RConn1 -- uac(+)/RConn1
  uac(-)/RConn1 -- full-bridge_ideal_switch_based/RConn2

== system sst_cllc_ttype_inv/dcdc_cllc_modA/dcdc_with_galvanic_isolation/full-bridge_2/full-bridge_mosfet_based_with_thermal_model ==
  gate_commands : Inport
  data_measure : Subsystem
  full-bridge_mosfet_based_with_thermal_model : full_bridge_mosfet_based_with_thermal_model/full-bridge mosfet based with thermal model  mass_heatsink_m=heatsink.no_weight  specific_heat_m=heatsink.cp  rth_mosfet_HA_m=heatsink.Rth_mosfet_HA  rth_mosfet_JH_m=mosfet.dab.Rth_mosfet_JH  Rds_on_m=mosfet.dab.Rds_on  Vth_m=mosfet.dab.Vth  Eon_m=mosfet.dab.Eon  Eoff_m=mosfet.dab.Eoff  Voff_sw_loss_m=mosfet.dab.Voff_sw_losses  Ion_sw_loss_m=mosfet.dab.Ion_sw_losses  Vdon_diode_m=mosfet.dab.Vdon_diode  Rdon_diode_m=mosfet.dab.Rds_on  JunctionTermalMass_m=mosfet.dab.JunctionTermalMass  Tambient_m=heatsink.Tambient  DThs_init_m=heatsink.DThs_init
  udc(+) : PMIOPort  Side=Left
  uac(+) : PMIOPort  Port=2  Side=Right
  udc(-) : PMIOPort  Port=3  Side=Left
  uac(-) : PMIOPort  Port=4  Side=Right
  wires:
  full-bridge_mosfet_based_with_thermal_model/1 -> data_measure/1(m)
  gate_commands/1 -> full-bridge_mosfet_based_with_thermal_model/1
  connections:
  full-bridge_mosfet_based_with_thermal_model/RConn2 -- uac(-)/RConn1
  full-bridge_mosfet_based_with_thermal_model/LConn1 -- udc(+)/RConn1
  udc(-)/RConn1 -- full-bridge_mosfet_based_with_thermal_model/LConn2
  full-bridge_mosfet_based_with_thermal_model/RConn1 -- uac(+)/RConn1

== system sst_cllc_ttype_inv/dcdc_cllc_modA/dcdc_with_galvanic_isolation/full-bridge_2/full-bridge_mosfet_based_with_thermal_model_zvs ==
  gate_commands : Inport
  data_measure : Subsystem
  full-bridge_mosfet_based_ with_thermal_model_zvs : full_bridge_mosfet_based_with_thermal_model_zvs/full-bridge_mosfet_based_ with_thermal_model_zvs  mass_heatsink_m=heatsink.no_weight  specific_heat_m=heatsink.cp  rth_mosfet_HA_m=heatsink.Rth_mosfet_HA  rth_mosfet_JH_m=mosfet.dab.Rth_mosfet_JH  Rds_on_m=mosfet.dab.Rds_on  Vth_m=mosfet.dab.Vth  Eon_m=mosfet.dab.Eon  Eoff_m=mosfet.dab.Eoff  Voff_sw_loss_m=mosfet.dab.Voff_sw_losses  Ion_sw_loss_m=mosfet.dab.Ion_sw_losses  Vdon_diode_m=mosfet.dab.Vdon_diode  Rdon_diode_m=mosfet.dab.Rds_on  JunctionTermalMass_m=mosfet.dab.JunctionTermalMass  Tambient_m=heatsink.Tambient  DThs_init_m=heatsink.DThs_init  Csnubber_m=mosfet.dab.Csnubber_zvs  Rsnubber_m=mosfet.dab.Rsnubber_zvs
  udc(+) : PMIOPort  Side=Left
  udc(-) : PMIOPort  Port=2  Side=Left
  uac(+) : PMIOPort  Port=3  Side=Right
  uac(-) : PMIOPort  Port=4  Side=Right
  wires:
  full-bridge_mosfet_based_ with_thermal_model_zvs/1 -> data_measure/1(m)
  gate_commands/1 -> full-bridge_mosfet_based_ with_thermal_model_zvs/1
  connections:
  full-bridge_mosfet_based_ with_thermal_model_zvs/LConn2 -- udc(-)/RConn1
  full-bridge_mosfet_based_ with_thermal_model_zvs/LConn1 -- udc(+)/RConn1
  full-bridge_mosfet_based_ with_thermal_model_zvs/RConn2 -- uac(-)/RConn1
  full-bridge_mosfet_based_ with_thermal_model_zvs/RConn1 -- uac(+)/RConn1

== system sst_cllc_ttype_inv/dcdc_cllc_modA/input_current_control/input_current_control/inner_ctrl ==
  i_ref : Inport
  i : Inport  Port=2
  current_control : Subsystem
  discrete-time-low-pass-filter : discrete_time_low_pass_filter/discrete-time-low-pass-filter  tau=500*glb_time.ts_cllc  ts=glb_time.ts_cllc
  discrete-time-low-pass-filter1 : discrete_time_low_pass_filter/discrete-time-low-pass-filter  tau=500*glb_time.ts_cllc  ts=glb_time.ts_cllc
  current_ctrl_output : Outport
  tag scope: current_ctrl_output=scoped, current_input_flt=scoped
  wires:
  current_control/1(ctrli_out) -> current_ctrl_output/1, [current_ctrl_output]  "current_ctrl_output"
  i_ref/1 -> current_control/1(i_ref)  "current_input_ref"
  i/1 -> [current_input_flt], current_control/2(i)  "current_input"

== system sst_cllc_ttype_inv/dcdc_cllc_modA/input_current_control/input_current_control/outer_ctrl ==
  u_ref : Inport
  u : Inport  Port=2
  current_control : Subsystem
  current_ctrl_output : Outport
  tag scope: voltage_control_output=scoped
  wires:
  current_control/1(ctrli_out) -> [voltage_control_output], current_ctrl_output/1  "voltage_ctrl_output"
  u_ref/1 -> current_control/1(iout_ref)  "u_ref"
  u/1 -> current_control/2(iout)  "u"

== system sst_cllc_ttype_inv/dcdc_cllc_modB/dcdc_with_galvanic_isolation/full-bridge_1/full-bridge_ideal_switch_based ==
  gate_commands : Inport
  data_measure : Subsystem
  full-bridge_ideal_switch_based : full_bridge_ideal_switch/full-bridge ideal switch based  Rds_on=ideal_switch.dab.Rds_on  Vdon_diode=ideal_switch.dab.Vdon_diode  Rdon_diode=ideal_switch.dab.Rdon_diode  Csnubber=ideal_switch.dab.Csnubber_zvs  Rsnubber=ideal_switch.dab.Rsnubber_zvs  Vth=ideal_switch.dab.Vth
  udc(+) : PMIOPort  Side=Left
  uac(+) : PMIOPort  Port=2  Side=Right
  udc(-) : PMIOPort  Port=3  Side=Left
  uac(-) : PMIOPort  Port=4  Side=Right
  wires:
  gate_commands/1 -> full-bridge_ideal_switch_based/1
  full-bridge_ideal_switch_based/1 -> data_measure/1(m)
  connections:
  uac(-)/RConn1 -- full-bridge_ideal_switch_based/RConn2
  full-bridge_ideal_switch_based/RConn1 -- uac(+)/RConn1
  udc(-)/RConn1 -- full-bridge_ideal_switch_based/LConn2
  udc(+)/RConn1 -- full-bridge_ideal_switch_based/LConn1

== system sst_cllc_ttype_inv/dcdc_cllc_modB/dcdc_with_galvanic_isolation/full-bridge_1/full-bridge_mosfet_based_with_thermal_model ==
  gate_commands : Inport
  data_measure : Subsystem
  full-bridge_mosfet_based_with_thermal_model : full_bridge_mosfet_based_with_thermal_model/full-bridge mosfet based with thermal model  mass_heatsink_m=heatsink.no_weight  specific_heat_m=heatsink.cp  rth_mosfet_HA_m=heatsink.Rth_mosfet_HA  rth_mosfet_JH_m=mosfet.dab.Rth_mosfet_JH  Rds_on_m=mosfet.dab.Rds_on  Vth_m=mosfet.dab.Vth  Eon_m=mosfet.dab.Eon  Eoff_m=mosfet.dab.Eoff  Voff_sw_loss_m=mosfet.dab.Voff_sw_losses  Ion_sw_loss_m=mosfet.dab.Ion_sw_losses  Vdon_diode_m=mosfet.dab.Vdon_diode  Rdon_diode_m=mosfet.dab.Rds_on  JunctionTermalMass_m=mosfet.dab.JunctionTermalMass  Tambient_m=heatsink.Tambient  DThs_init_m=heatsink.DThs_init
  udc(+) : PMIOPort  Side=Left
  uac(+) : PMIOPort  Port=2  Side=Right
  udc(-) : PMIOPort  Port=3  Side=Left
  uac(-) : PMIOPort  Port=4  Side=Right
  wires:
  gate_commands/1 -> full-bridge_mosfet_based_with_thermal_model/1
  full-bridge_mosfet_based_with_thermal_model/1 -> data_measure/1(m)
  connections:
  full-bridge_mosfet_based_with_thermal_model/RConn1 -- uac(+)/RConn1
  udc(-)/RConn1 -- full-bridge_mosfet_based_with_thermal_model/LConn2
  full-bridge_mosfet_based_with_thermal_model/LConn1 -- udc(+)/RConn1
  full-bridge_mosfet_based_with_thermal_model/RConn2 -- uac(-)/RConn1

== system sst_cllc_ttype_inv/dcdc_cllc_modB/dcdc_with_galvanic_isolation/full-bridge_1/full-bridge_mosfet_based_with_thermal_model_zvs ==
  gate_commands : Inport
  data_measure : Subsystem
  full-bridge_mosfet_based_ with_thermal_model_zvs : full_bridge_mosfet_based_with_thermal_model_zvs/full-bridge_mosfet_based_ with_thermal_model_zvs  mass_heatsink_m=heatsink.no_weight  specific_heat_m=heatsink.cp  rth_mosfet_HA_m=heatsink.Rth_mosfet_HA  rth_mosfet_JH_m=mosfet.dab.Rth_mosfet_JH  Rds_on_m=mosfet.dab.Rds_on  Vth_m=mosfet.dab.Vth  Eon_m=mosfet.dab.Eon  Eoff_m=mosfet.dab.Eoff  Voff_sw_loss_m=mosfet.dab.Voff_sw_losses  Ion_sw_loss_m=mosfet.dab.Ion_sw_losses  Vdon_diode_m=mosfet.dab.Vdon_diode  Rdon_diode_m=mosfet.dab.Rds_on  JunctionTermalMass_m=mosfet.dab.JunctionTermalMass  Tambient_m=heatsink.Tambient  DThs_init_m=heatsink.DThs_init  Csnubber_m=mosfet.dab.Csnubber_zvs  Rsnubber_m=mosfet.dab.Rsnubber_zvs
  udc(+) : PMIOPort  Side=Left
  udc(-) : PMIOPort  Port=2  Side=Left
  uac(+) : PMIOPort  Port=3  Side=Right
  uac(-) : PMIOPort  Port=4  Side=Right
  wires:
  gate_commands/1 -> full-bridge_mosfet_based_ with_thermal_model_zvs/1
  full-bridge_mosfet_based_ with_thermal_model_zvs/1 -> data_measure/1(m)
  connections:
  full-bridge_mosfet_based_ with_thermal_model_zvs/RConn1 -- uac(+)/RConn1
  full-bridge_mosfet_based_ with_thermal_model_zvs/RConn2 -- uac(-)/RConn1
  full-bridge_mosfet_based_ with_thermal_model_zvs/LConn1 -- udc(+)/RConn1
  full-bridge_mosfet_based_ with_thermal_model_zvs/LConn2 -- udc(-)/RConn1

== system sst_cllc_ttype_inv/dcdc_cllc_modB/dcdc_with_galvanic_isolation/full-bridge_2/full-bridge_ideal_switch_based ==
  gate_commands : Inport
  data_measure : Subsystem
  full-bridge_ideal_switch_based : full_bridge_ideal_switch/full-bridge ideal switch based  Rds_on=ideal_switch.dab.Rds_on  Vdon_diode=ideal_switch.dab.Vdon_diode  Rdon_diode=ideal_switch.dab.Rdon_diode  Csnubber=ideal_switch.dab.Csnubber_zvs  Rsnubber=ideal_switch.dab.Rsnubber_zvs  Vth=ideal_switch.dab.Vth
  udc(+) : PMIOPort  Side=Left
  uac(+) : PMIOPort  Port=2  Side=Right
  udc(-) : PMIOPort  Port=3  Side=Left
  uac(-) : PMIOPort  Port=4  Side=Right
  wires:
  gate_commands/1 -> full-bridge_ideal_switch_based/1
  full-bridge_ideal_switch_based/1 -> data_measure/1(m)
  connections:
  uac(-)/RConn1 -- full-bridge_ideal_switch_based/RConn2
  full-bridge_ideal_switch_based/RConn1 -- uac(+)/RConn1
  udc(-)/RConn1 -- full-bridge_ideal_switch_based/LConn2
  udc(+)/RConn1 -- full-bridge_ideal_switch_based/LConn1

== system sst_cllc_ttype_inv/dcdc_cllc_modB/dcdc_with_galvanic_isolation/full-bridge_2/full-bridge_mosfet_based_with_thermal_model ==
  gate_commands : Inport
  data_measure : Subsystem
  full-bridge_mosfet_based_with_thermal_model : full_bridge_mosfet_based_with_thermal_model/full-bridge mosfet based with thermal model  mass_heatsink_m=heatsink.no_weight  specific_heat_m=heatsink.cp  rth_mosfet_HA_m=heatsink.Rth_mosfet_HA  rth_mosfet_JH_m=mosfet.dab.Rth_mosfet_JH  Rds_on_m=mosfet.dab.Rds_on  Vth_m=mosfet.dab.Vth  Eon_m=mosfet.dab.Eon  Eoff_m=mosfet.dab.Eoff  Voff_sw_loss_m=mosfet.dab.Voff_sw_losses  Ion_sw_loss_m=mosfet.dab.Ion_sw_losses  Vdon_diode_m=mosfet.dab.Vdon_diode  Rdon_diode_m=mosfet.dab.Rds_on  JunctionTermalMass_m=mosfet.dab.JunctionTermalMass  Tambient_m=heatsink.Tambient  DThs_init_m=heatsink.DThs_init
  udc(+) : PMIOPort  Side=Left
  uac(+) : PMIOPort  Port=2  Side=Right
  udc(-) : PMIOPort  Port=3  Side=Left
  uac(-) : PMIOPort  Port=4  Side=Right
  wires:
  gate_commands/1 -> full-bridge_mosfet_based_with_thermal_model/1
  full-bridge_mosfet_based_with_thermal_model/1 -> data_measure/1(m)
  connections:
  full-bridge_mosfet_based_with_thermal_model/RConn1 -- uac(+)/RConn1
  udc(-)/RConn1 -- full-bridge_mosfet_based_with_thermal_model/LConn2
  full-bridge_mosfet_based_with_thermal_model/LConn1 -- udc(+)/RConn1
  full-bridge_mosfet_based_with_thermal_model/RConn2 -- uac(-)/RConn1

== system sst_cllc_ttype_inv/dcdc_cllc_modB/dcdc_with_galvanic_isolation/full-bridge_2/full-bridge_mosfet_based_with_thermal_model_zvs ==
  gate_commands : Inport
  data_measure : Subsystem
  full-bridge_mosfet_based_ with_thermal_model_zvs : full_bridge_mosfet_based_with_thermal_model_zvs/full-bridge_mosfet_based_ with_thermal_model_zvs  mass_heatsink_m=heatsink.no_weight  specific_heat_m=heatsink.cp  rth_mosfet_HA_m=heatsink.Rth_mosfet_HA  rth_mosfet_JH_m=mosfet.dab.Rth_mosfet_JH  Rds_on_m=mosfet.dab.Rds_on  Vth_m=mosfet.dab.Vth  Eon_m=mosfet.dab.Eon  Eoff_m=mosfet.dab.Eoff  Voff_sw_loss_m=mosfet.dab.Voff_sw_losses  Ion_sw_loss_m=mosfet.dab.Ion_sw_losses  Vdon_diode_m=mosfet.dab.Vdon_diode  Rdon_diode_m=mosfet.dab.Rds_on  JunctionTermalMass_m=mosfet.dab.JunctionTermalMass  Tambient_m=heatsink.Tambient  DThs_init_m=heatsink.DThs_init  Csnubber_m=mosfet.dab.Csnubber_zvs  Rsnubber_m=mosfet.dab.Rsnubber_zvs
  udc(+) : PMIOPort  Side=Left
  udc(-) : PMIOPort  Port=2  Side=Left
  uac(+) : PMIOPort  Port=3  Side=Right
  uac(-) : PMIOPort  Port=4  Side=Right
  wires:
  gate_commands/1 -> full-bridge_mosfet_based_ with_thermal_model_zvs/1
  full-bridge_mosfet_based_ with_thermal_model_zvs/1 -> data_measure/1(m)
  connections:
  full-bridge_mosfet_based_ with_thermal_model_zvs/RConn1 -- uac(+)/RConn1
  full-bridge_mosfet_based_ with_thermal_model_zvs/RConn2 -- uac(-)/RConn1
  full-bridge_mosfet_based_ with_thermal_model_zvs/LConn1 -- udc(+)/RConn1
  full-bridge_mosfet_based_ with_thermal_model_zvs/LConn2 -- udc(-)/RConn1

== system sst_cllc_ttype_inv/dcdc_cllc_modB/input_current_control/input_current_control/inner_ctrl ==
  i_ref : Inport
  i : Inport  Port=2
  current_control : Subsystem
  discrete-time-low-pass-filter : discrete_time_low_pass_filter/discrete-time-low-pass-filter  tau=500*glb_time.ts_cllc  ts=glb_time.ts_cllc
  discrete-time-low-pass-filter1 : discrete_time_low_pass_filter/discrete-time-low-pass-filter  tau=500*glb_time.ts_cllc  ts=glb_time.ts_cllc
  current_ctrl_output : Outport
  tag scope: current_ctrl_output=scoped, current_input_flt=scoped
  wires:
  i/1 -> current_control/2(i), [current_input_flt]  "current_input"
  current_control/1(ctrli_out) -> [current_ctrl_output], current_ctrl_output/1  "current_ctrl_output"
  i_ref/1 -> current_control/1(i_ref)  "current_input_ref"

== system sst_cllc_ttype_inv/dcdc_cllc_modB/input_current_control/input_current_control/outer_ctrl ==
  u_ref : Inport
  u : Inport  Port=2
  current_control : Subsystem
  current_ctrl_output : Outport
  tag scope: voltage_control_output=scoped
  wires:
  u/1 -> current_control/2(iout)  "u"
  u_ref/1 -> current_control/1(iout_ref)  "u_ref"
  current_control/1(ctrli_out) -> current_ctrl_output/1, [voltage_control_output]  "voltage_ctrl_output"
